simulink model "Simulink"  (R2022b)
settings: Solver=VariableStepAuto  StartTime=0.0  StopTime=3  RelTol=1e-3
values from neighbouring files (symbols this model uses):
  ASim = A    [Assignment1.m]
  BSim = B    [Assignment1.m]
  C1Sim = C1    [Assignment1.m]
  C2Sim = C2    [Assignment1.m]
  D1Sim = D1    (= 20)    [Assignment1.m]
  D2Sim = D2    (= 2)    [Assignment1.m]
settings Model: Creator=aksha  LastModifiedBy=aksha
settings ModelReferenceCC: EnableRefExpFcnMdlSchedulingChecks=on

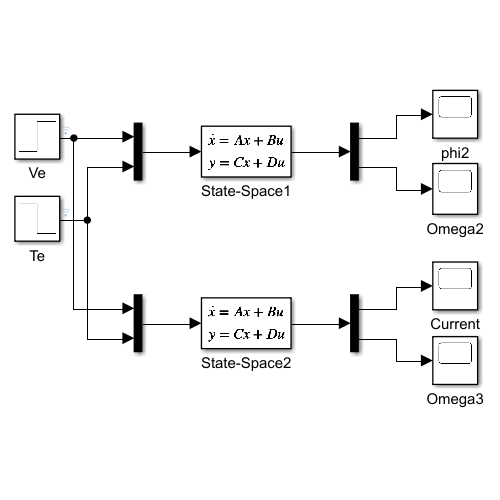
[thumbnail: Simulink's stored preview of the top-level diagram]
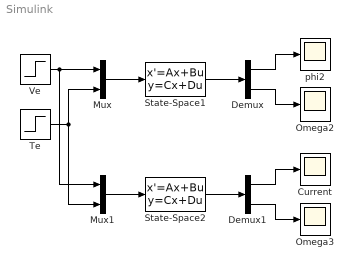
== system Simulink ==
  Current : Scope
  Demux : Demux  Outputs=2
  Demux1 : Demux  Outputs=2
  Mux : Mux  Inputs=2
  Mux1 : Mux  Inputs=2
  Omega2 : Scope
  Omega3 : Scope
  State-Space1 : StateSpace  A=ASim  B=BSim  C=C1Sim  D=D1Sim  InitialCondition=0  AllowTunableDMatrix=on
  State-Space2 : StateSpace  A=ASim  B=BSim  C=C2Sim  D=D2Sim  InitialCondition=0  AllowTunableDMatrix=on
  Te : Step  After=-0.1  SampleTime=0
  Ve : Step  Time=0.2  After=10  SampleTime=0
  phi2 : Scope
  wires:
  Mux/1 -> State-Space1/1
  State-Space1/1 -> Demux/1
  Demux/1 -> phi2/1
  Demux/2 -> Omega2/1
  Te/1 -> Mux/2, Mux1/2
  Mux1/1 -> State-Space2/1
  Demux1/1 -> Current/1
  Ve/1 -> Mux/1, Mux1/1
  Demux1/2 -> Omega3/1
  State-Space2/1 -> Demux1/1
